simulink model "cactinhchatpho"  (Simulink 7.3)
settings: Solver=ode45  StartTime=0.0  StopTime=1  RelTol=1e-3
libraries: simulink x1
settings Model: Creator=nthuy  LastModifiedBy=nthuy

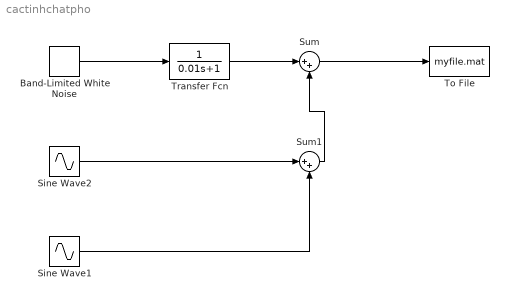
== system cactinhchatpho ==
  Band-Limited White Noise : simulink/Sources/Band-Limited White Noise  SystemSampleTime=-1  Cov=[0.01]  Ts=0.001  seed=[23341]
  Sine Wave1 : Sin  Amplitude=1  Bias=0  Frequency=2*pi*220  Phase=0  Samples=10  SampleTime=0  Offset=0
  Sine Wave2 : Sin  Amplitude=1  Bias=0  Frequency=2*pi*200  Phase=0  Samples=10  SampleTime=0  Offset=0
  Sum : Sum  Inputs=|++  OutDataType=fixdt(1, 16)  OutScaling=2^0
  Sum1 : Sum  Inputs=|++  OutDataType=fixdt(1, 16)  OutScaling=2^0
  To File : ToFile  Filename=myfile.mat  MatrixName=xx  SampleTime=0.001
  Transfer Fcn : TransferFcn  Denominator=[0.01 1]
  wires:
  Band-Limited White Noise/1 -> Transfer Fcn/1
  Transfer Fcn/1 -> Sum/1
  Sine Wave2/1 -> Sum1/1
  Sine Wave1/1 -> Sum1/2
  Sum1/1 -> Sum/2
  Sum/1 -> To File/1
